simulink model "ped_pr7_120conductionmode"  (R2023b)
settings: Solver=VariableStepAuto  StartTime=0.0  StopTime=10.0  RelTol=1e-3
libraries: spsMosfetLib x6, spsRMSLib x2, spsVoltageMeasurementLib x2, spsDCVoltageSourceLib x1, spsGroundLib x1, spsThreePhaseSeriesRLCLoadLib x1, sps_lib x1
settings Model: Creator=vaish  LastModifiedBy=vaish

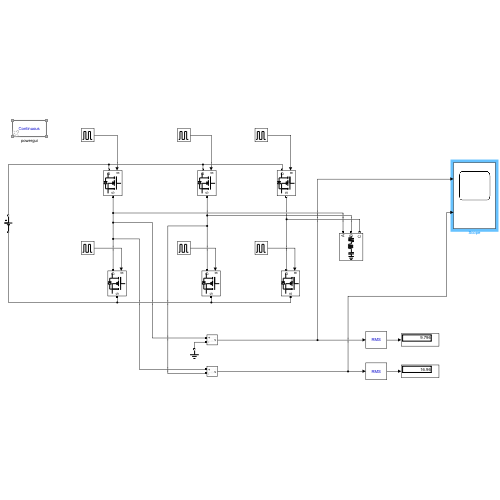
[thumbnail: Simulink's stored preview of the top-level diagram]
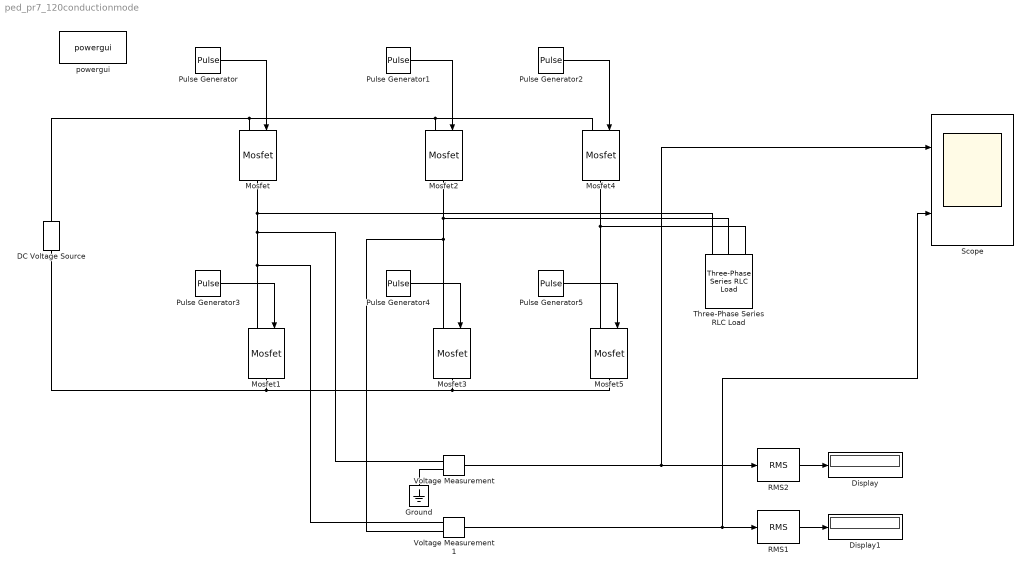
== system ped_pr7_120conductionmode ==
  DC Voltage Source : spsDCVoltageSourceLib/DC Voltage Source  Amplitude=24  Measurements=None
  Display : Display
  Display1 : Display
  Ground : spsGroundLib/Ground  LConnTagsString=a
  Mosfet{,1..5} (6 alike) : spsMosfetLib/Mosfet  Ron=0.1  Lon=0  Rd=0.01  Vfd=0  IC=0  Rs=1e5  Cs=inf  Measurements=off
  Pulse Generator : DiscretePulseGenerator  PulseType=Time based  Period=0.02  PulseWidth=33.33
  Pulse Generator1 : DiscretePulseGenerator  PulseType=Time based  Period=0.02  PulseWidth=33.33  PhaseDelay=0.00666
  Pulse Generator2 : DiscretePulseGenerator  PulseType=Time based  Period=0.02  PulseWidth=33.33  PhaseDelay=0.01332
  Pulse Generator3 : DiscretePulseGenerator  PulseType=Time based  Period=0.02  PulseWidth=33.33  PhaseDelay=0.00999
  Pulse Generator4 : DiscretePulseGenerator  PulseType=Time based  Period=0.02  PulseWidth=33.33  PhaseDelay=0.01665
  Pulse Generator5 : DiscretePulseGenerator  PulseType=Time based  Period=0.02  PulseWidth=33.33  PhaseDelay=0.00333
  RMS1 : spsRMSLib/RMS  TrueRMS=on  Freq=50  RMSInit=120  Ts=0
  RMS2 : spsRMSLib/RMS  TrueRMS=on  Freq=50  RMSInit=120  Ts=0
  Scope : Scope  NumInputPorts=2
  Three-Phase Series RLC Load : spsThreePhaseSeriesRLCLoadLib/Three-Phase Series RLC Load  LConnTagsString=A|B|C  Configuration=Y (grounded)  NominalVoltage=1000  Vabc=[1e3 1e3 1e3]  Vabcp=[1e3 1e3 1e3]  NominalFrequency=60  UnbalancedPower=off  ActivePower=10e3  InductivePower=100  CapacitivePower=100  Pabc=[10e3 9e3 11e3]  QLabc=[100 90 110]  QCabc=[100 90 110]  Pabcp=[10e3 9e3 11e3]  QLabcp=[100 90 110]  QCabcp=[100 90 110]  Measurements=None  LoadType=constant Z
  Voltage Measurement : spsVoltageMeasurementLib/Voltage Measurement  PhasorSimulation=off  OutputType=Complex  PSBequivalent=0
  Voltage Measurement1 : spsVoltageMeasurementLib/Voltage Measurement  PhasorSimulation=off  OutputType=Complex  PSBequivalent=0
  powergui : sps_lib/powergui  Priority=1  SimulationMode=Continuous  SampleTime=50e-6  frequency=60  Iterations=50  frequencyindice=0  Pbase=100e6  ErrMax=1e-4  UnitsV=kV  UnitsW=MW  buscounter=0  FunctionMessages=off  echomessages=off  EnableUseOfTLC=off  CurrentSourceSwitches=off  DisableSnubberDevices=off  DisableRonSwitches=off  DisableVfSwitches=off  DisplayEquations=off  AutomaticDiscreteSolvers=off  SolverType=Tustin/Backward Euler (TBE)  Interpol=off  ExternalGateDelay=off  methode=off  Ts=100  x0status=blocks  SPID=on  SwTol=0  HookPort=off  NonlinearTolerance=1e-4  nMaxIteration=100  ContinueOnMaxIteration=off  RestoreLinks=warning  ResistiveCurrentMeasurement=off  Frange=[0:2:500]  Ylog=off  Xlog=on  ShowGrid=off  save=off  variable=ZData  structure=0  ZoomFFT=off  StartTime=0.0  cycles=1  DisplayStyle=1  fundamental=60  FreqAxis=off  MaxFrequency=1000  frequencyindicesteady=1  RmsSteady=1  display=off
  wires:
  Voltage Measurement/1 -> Scope/1, RMS2/1
  Pulse Generator/1 -> Mosfet/1
  Pulse Generator4/1 -> Mosfet3/1
  Pulse Generator1/1 -> Mosfet2/1
  Pulse Generator5/1 -> Mosfet5/1
  Pulse Generator3/1 -> Mosfet1/1
  Voltage Measurement1/1 -> Scope/2, RMS1/1
  RMS1/1 -> Display1/1
  Pulse Generator2/1 -> Mosfet4/1
  RMS2/1 -> Display/1
  connections:
  Mosfet2/LConn1 -- Mosfet4/LConn1 -- Mosfet/LConn1 -- DC Voltage Source/RConn1
  Mosfet3/RConn1 -- Mosfet5/RConn1 -- DC Voltage Source/LConn1 -- Mosfet1/RConn1
  Mosfet2/RConn1 -- Three-Phase Series RLC Load/LConn2 -- Mosfet3/LConn1 -- Voltage Measurement1/LConn2
  Mosfet/RConn1 -- Three-Phase Series RLC Load/LConn1 -- Voltage Measurement/LConn1 -- Voltage Measurement1/LConn1 -- Mosfet1/LConn1
  Mosfet5/LConn1 -- Three-Phase Series RLC Load/LConn3 -- Mosfet4/RConn1
  Ground/LConn1 -- Voltage Measurement/LConn2
